simulink model "aes_impl_decrypt_smc"  (R2015b)
settings: Solver=FixedStepDiscrete  SolverMode=SingleTasking  StartTime=0.0  StopTime=1000e-6  RelTol=1e-3
undefined symbols (not defined in the file): a, b, input_sample_rate
libraries: shlslibv1 x3018
(part 4 of 20)

== system aes_impl_decrypt_smc/Round12/Subsystem8 ==
  In1 : Inport
  In2 : Inport  Port=2
  In3 : Inport  Port=3
  In4 : Inport  Port=4
  In5 : Inport  Port=5
  In6 : Inport  Port=6
  In7 : Inport  Port=7
  In8 : Inport  Port=8
  In9 : Inport  Port=9
  In10 : Inport  Port=10
  In11 : Inport  Port=11
  In12 : Inport  Port=12
  In13 : Inport  Port=13
  In14 : Inport  Port=14
  In15 : Inport  Port=15
  In16 : Inport  Port=16
  Subsystem : Subsystem
  Subsystem1 : Subsystem
  Subsystem2 : Subsystem
  Subsystem3 : Subsystem
  Subsystem4 : Subsystem
  Subsystem5 : Subsystem
  Subsystem6 : Subsystem
  Subsystem7 : Subsystem
  Subsystem8 : Subsystem
  Out1 : Outport
  Out2 : Outport  Port=2
  Out3 : Outport  Port=3
  Out4 : Outport  Port=4
  Out5 : Outport  Port=5
  Out6 : Outport  Port=6
  Out7 : Outport  Port=7
  Out8 : Outport  Port=8
  Out9 : Outport  Port=9
  Out10 : Outport  Port=10
  Out11 : Outport  Port=11
  Out12 : Outport  Port=12
  Out13 : Outport  Port=13
  Out14 : Outport  Port=14
  Out15 : Outport  Port=15
  Out16 : Outport  Port=16
  wires:
  Subsystem4/3(Out3) -> Out3/1
  Subsystem4/4(Out4) -> Out4/1
  Subsystem1/1(Out1) -> Out5/1
  Subsystem1/2(Out2) -> Out6/1
  Subsystem1/3(Out3) -> Out7/1
  Subsystem1/4(Out4) -> Out8/1
  Subsystem2/3(Out3) -> Out11/1
  Subsystem2/2(Out2) -> Out10/1
  Subsystem2/1(Out1) -> Out9/1
  Subsystem2/4(Out4) -> Out12/1
  Subsystem3/3(Out3) -> Out15/1
  Subsystem3/2(Out2) -> Out14/1
  Subsystem3/1(Out1) -> Out13/1
  Subsystem/1(Out1) -> Subsystem4/1(In1)
  Subsystem/2(Out2) -> Subsystem4/2(In2)
  Subsystem/3(Out3) -> Subsystem4/3(In3)
  Subsystem/4(Out4) -> Subsystem4/4(In4)
  Subsystem/5(Out5) -> Subsystem1/1(In1)
  Subsystem/6(Out6) -> Subsystem1/2(In2)
  Subsystem/7(Out7) -> Subsystem1/3(In3)
  Subsystem/8(Out8) -> Subsystem1/4(In4)
  Subsystem/9(Out9) -> Subsystem2/1(In1)
  Subsystem/10(Out10) -> Subsystem2/2(In2)
  Subsystem/11(Out11) -> Subsystem2/3(In3)
  Subsystem/12(Out12) -> Subsystem2/4(In4)
  Subsystem/14(Out14) -> Subsystem3/2(In2)
  Subsystem4/1(Out1) -> Out1/1
  Subsystem4/2(Out2) -> Out2/1
  Subsystem3/4(Out4) -> Out16/1
  Subsystem/13(Out13) -> Subsystem3/1(In1)
  Subsystem/15(Out15) -> Subsystem3/3(In3)
  Subsystem/16(Out16) -> Subsystem3/4(In4)
  Subsystem5/2(Out18) -> Subsystem/2(In2)
  Subsystem5/1(Out17) -> Subsystem/1(In1)
  Subsystem5/3(Out19) -> Subsystem/3(In3)
  Subsystem5/4(Out20) -> Subsystem/4(In4)
  In1/1 -> Subsystem5/1(In17)
  In2/1 -> Subsystem5/2(In18)
  In3/1 -> Subsystem5/3(In19)
  In4/1 -> Subsystem5/4(In20)
  Subsystem6/2(Out18) -> Subsystem/6(In6)
  Subsystem6/1(Out17) -> Subsystem/5(In5)
  Subsystem6/3(Out19) -> Subsystem/7(In7)
  Subsystem6/4(Out20) -> Subsystem/8(In8)
  In5/1 -> Subsystem6/1(In17)
  In6/1 -> Subsystem6/2(In18)
  In7/1 -> Subsystem6/3(In19)
  In8/1 -> Subsystem6/4(In20)
  Subsystem7/2(Out18) -> Subsystem/10(In10)
  Subsystem7/1(Out17) -> Subsystem/9(In9)
  Subsystem7/3(Out19) -> Subsystem/11(In11)
  Subsystem7/4(Out20) -> Subsystem/12(In12)
  In9/1 -> Subsystem7/1(In17)
  In10/1 -> Subsystem7/2(In18)
  In11/1 -> Subsystem7/3(In19)
  In12/1 -> Subsystem7/4(In20)
  Subsystem8/2(Out18) -> Subsystem/14(In14)
  Subsystem8/1(Out17) -> Subsystem/13(In13)
  Subsystem8/3(Out19) -> Subsystem/15(In15)
  Subsystem8/4(Out20) -> Subsystem/16(In16)
  In13/1 -> Subsystem8/1(In17)
  In14/1 -> Subsystem8/2(In18)
  In15/1 -> Subsystem8/3(In19)
  In16/1 -> Subsystem8/4(In20)

== system aes_impl_decrypt_smc/Round13/Subsystem ==
  In1 : Inport
  In2 : Inport  Port=2
  In3 : Inport  Port=3
  In4 : Inport  Port=4
  In5 : Inport  Port=5
  In6 : Inport  Port=6
  In7 : Inport  Port=7
  In8 : Inport  Port=8
  In9 : Inport  Port=9
  In10 : Inport  Port=10
  In11 : Inport  Port=11
  In12 : Inport  Port=12
  In13 : Inport  Port=13
  In14 : Inport  Port=14
  In15 : Inport  Port=15
  In16 : Inport  Port=16
  In17 : Inport  Port=17
  In18 : Inport  Port=18
  In19 : Inport  Port=19
  In20 : Inport  Port=20
  In21 : Inport  Port=21
  In22 : Inport  Port=22
  In23 : Inport  Port=23
  In24 : Inport  Port=24
  In25 : Inport  Port=25
  In26 : Inport  Port=26
  In27 : Inport  Port=27
  In28 : Inport  Port=28
  In29 : Inport  Port=29
  In30 : Inport  Port=30
  In31 : Inport  Port=31
  In32 : Inport  Port=32
  Binary Logic{,1..15} (16 alike) : shlslibv1/Math Functions/Binary Logic  syn_binlog_exp=a^b  synBlockType=primitive  synLatency=0  synBlockId=13
  Out1 : Outport
  Out2 : Outport  Port=2
  Out3 : Outport  Port=3
  Out4 : Outport  Port=4
  Out5 : Outport  Port=5
  Out6 : Outport  Port=6
  Out7 : Outport  Port=7
  Out8 : Outport  Port=8
  Out9 : Outport  Port=9
  Out10 : Outport  Port=10
  Out11 : Outport  Port=11
  Out12 : Outport  Port=12
  Out13 : Outport  Port=13
  Out14 : Outport  Port=14
  Out15 : Outport  Port=15
  Out16 : Outport  Port=16
  wires:
  In9/1 -> Binary Logic8/1
  In11/1 -> Binary Logic10/1
  In8/1 -> Binary Logic7/1
  In16/1 -> Binary Logic15/1
  In3/1 -> Binary Logic2/1
  In12/1 -> Binary Logic11/1
  In10/1 -> Binary Logic9/1
  In13/1 -> Binary Logic12/1
  In15/1 -> Binary Logic14/1
  In14/1 -> Binary Logic13/1
  In7/1 -> Binary Logic6/1
  In6/1 -> Binary Logic5/1
  Binary Logic/1 -> Out1/1
  In4/1 -> Binary Logic3/1
  In5/1 -> Binary Logic4/1
  In2/1 -> Binary Logic1/1
  In18/1 -> Binary Logic1/2
  In19/1 -> Binary Logic2/2
  In20/1 -> Binary Logic3/2
  In21/1 -> Binary Logic4/2
  In22/1 -> Binary Logic5/2
  In23/1 -> Binary Logic6/2
  In24/1 -> Binary Logic7/2
  In25/1 -> Binary Logic8/2
  In26/1 -> Binary Logic9/2
  In27/1 -> Binary Logic10/2
  In28/1 -> Binary Logic11/2
  In29/1 -> Binary Logic12/2
  In30/1 -> Binary Logic13/2
  In31/1 -> Binary Logic14/2
  In32/1 -> Binary Logic15/2
  In1/1 -> Binary Logic/1
  In17/1 -> Binary Logic/2
  Binary Logic1/1 -> Out2/1
  Binary Logic2/1 -> Out3/1
  Binary Logic3/1 -> Out4/1
  Binary Logic4/1 -> Out5/1
  Binary Logic5/1 -> Out6/1
  Binary Logic6/1 -> Out7/1
  Binary Logic7/1 -> Out8/1
  Binary Logic8/1 -> Out9/1
  Binary Logic9/1 -> Out10/1
  Binary Logic15/1 -> Out16/1
  Binary Logic14/1 -> Out15/1
  Binary Logic13/1 -> Out14/1
  Binary Logic12/1 -> Out13/1
  Binary Logic11/1 -> Out12/1
  Binary Logic10/1 -> Out11/1

== system aes_impl_decrypt_smc/Round13/Subsystem8 ==
  In1 : Inport
  In2 : Inport  Port=2
  In3 : Inport  Port=3
  In4 : Inport  Port=4
  In5 : Inport  Port=5
  In6 : Inport  Port=6
  In7 : Inport  Port=7
  In8 : Inport  Port=8
  In9 : Inport  Port=9
  In10 : Inport  Port=10
  In11 : Inport  Port=11
  In12 : Inport  Port=12
  In13 : Inport  Port=13
  In14 : Inport  Port=14
  In15 : Inport  Port=15
  In16 : Inport  Port=16
  Subsystem : Subsystem
  Subsystem1 : Subsystem
  Subsystem2 : Subsystem
  Subsystem3 : Subsystem
  Subsystem4 : Subsystem
  Out1 : Outport
  Out2 : Outport  Port=2
  Out3 : Outport  Port=3
  Out4 : Outport  Port=4
  Out5 : Outport  Port=5
  Out6 : Outport  Port=6
  Out7 : Outport  Port=7
  Out8 : Outport  Port=8
  Out9 : Outport  Port=9
  Out10 : Outport  Port=10
  Out11 : Outport  Port=11
  Out12 : Outport  Port=12
  Out13 : Outport  Port=13
  Out14 : Outport  Port=14
  Out15 : Outport  Port=15
  Out16 : Outport  Port=16
  wires:
  Subsystem4/3(Out3) -> Out3/1
  Subsystem4/4(Out4) -> Out4/1
  Subsystem1/1(Out1) -> Out5/1
  Subsystem1/2(Out2) -> Out6/1
  Subsystem1/3(Out3) -> Out7/1
  Subsystem1/4(Out4) -> Out8/1
  Subsystem2/3(Out3) -> Out11/1
  Subsystem2/2(Out2) -> Out10/1
  Subsystem2/1(Out1) -> Out9/1
  Subsystem2/4(Out4) -> Out12/1
  Subsystem3/3(Out3) -> Out15/1
  Subsystem3/2(Out2) -> Out14/1
  Subsystem3/1(Out1) -> Out13/1
  In1/1 -> Subsystem/1(In1)
  In2/1 -> Subsystem/2(In2)
  In3/1 -> Subsystem/3(In3)
  In4/1 -> Subsystem/4(In4)
  In5/1 -> Subsystem/5(In5)
  In6/1 -> Subsystem/6(In6)
  In7/1 -> Subsystem/7(In7)
  In8/1 -> Subsystem/8(In8)
  In9/1 -> Subsystem/9(In9)
  In10/1 -> Subsystem/10(In10)
  In11/1 -> Subsystem/11(In11)
  In12/1 -> Subsystem/12(In12)
  In13/1 -> Subsystem/13(In13)
  In14/1 -> Subsystem/14(In14)
  In15/1 -> Subsystem/15(In15)
  In16/1 -> Subsystem/16(In16)
  Subsystem/1(Out1) -> Subsystem4/1(In1)
  Subsystem/2(Out2) -> Subsystem4/2(In2)
  Subsystem/3(Out3) -> Subsystem4/3(In3)
  Subsystem/4(Out4) -> Subsystem4/4(In4)
  Subsystem/5(Out5) -> Subsystem1/1(In1)
  Subsystem/6(Out6) -> Subsystem1/2(In2)
  Subsystem/7(Out7) -> Subsystem1/3(In3)
  Subsystem/8(Out8) -> Subsystem1/4(In4)
  Subsystem/9(Out9) -> Subsystem2/1(In1)
  Subsystem/10(Out10) -> Subsystem2/2(In2)
  Subsystem/11(Out11) -> Subsystem2/3(In3)
  Subsystem/12(Out12) -> Subsystem2/4(In4)
  Subsystem/14(Out14) -> Subsystem3/2(In2)
  Subsystem4/1(Out1) -> Out1/1
  Subsystem4/2(Out2) -> Out2/1
  Subsystem3/4(Out4) -> Out16/1
  Subsystem/13(Out13) -> Subsystem3/1(In1)
  Subsystem/15(Out15) -> Subsystem3/3(In3)
  Subsystem/16(Out16) -> Subsystem3/4(In4)

== system aes_impl_decrypt_smc/Round14/Subsystem ==
  In1 : Inport
  In2 : Inport  Port=2
  In3 : Inport  Port=3
  In4 : Inport  Port=4
  In5 : Inport  Port=5
  In6 : Inport  Port=6
  In7 : Inport  Port=7
  In8 : Inport  Port=8
  In9 : Inport  Port=9
  In10 : Inport  Port=10
  In11 : Inport  Port=11
  In12 : Inport  Port=12
  In13 : Inport  Port=13
  In14 : Inport  Port=14
  In15 : Inport  Port=15
  In16 : Inport  Port=16
  In17 : Inport  Port=17
  In18 : Inport  Port=18
  In19 : Inport  Port=19
  In20 : Inport  Port=20
  In21 : Inport  Port=21
  In22 : Inport  Port=22
  In23 : Inport  Port=23
  In24 : Inport  Port=24
  In25 : Inport  Port=25
  In26 : Inport  Port=26
  In27 : Inport  Port=27
  In28 : Inport  Port=28
  In29 : Inport  Port=29
  In30 : Inport  Port=30
  In31 : Inport  Port=31
  In32 : Inport  Port=32
  Binary Logic{,1..15} (16 alike) : shlslibv1/Math Functions/Binary Logic  syn_binlog_exp=a^b  synBlockType=primitive  synLatency=0  synBlockId=13
  Out1 : Outport
  Out2 : Outport  Port=2
  Out3 : Outport  Port=3
  Out4 : Outport  Port=4
  Out5 : Outport  Port=5
  Out6 : Outport  Port=6
  Out7 : Outport  Port=7
  Out8 : Outport  Port=8
  Out9 : Outport  Port=9
  Out10 : Outport  Port=10
  Out11 : Outport  Port=11
  Out12 : Outport  Port=12
  Out13 : Outport  Port=13
  Out14 : Outport  Port=14
  Out15 : Outport  Port=15
  Out16 : Outport  Port=16
  wires:
  In9/1 -> Binary Logic8/1
  In11/1 -> Binary Logic10/1
  In8/1 -> Binary Logic7/1
  In16/1 -> Binary Logic15/1
  In3/1 -> Binary Logic2/1
  In12/1 -> Binary Logic11/1
  In10/1 -> Binary Logic9/1
  In13/1 -> Binary Logic12/1
  In15/1 -> Binary Logic14/1
  In14/1 -> Binary Logic13/1
  In7/1 -> Binary Logic6/1
  In6/1 -> Binary Logic5/1
  Binary Logic/1 -> Out1/1
  In4/1 -> Binary Logic3/1
  In5/1 -> Binary Logic4/1
  In2/1 -> Binary Logic1/1
  In18/1 -> Binary Logic1/2
  In19/1 -> Binary Logic2/2
  In20/1 -> Binary Logic3/2
  In21/1 -> Binary Logic4/2
  In22/1 -> Binary Logic5/2
  In23/1 -> Binary Logic6/2
  In24/1 -> Binary Logic7/2
  In25/1 -> Binary Logic8/2
  In26/1 -> Binary Logic9/2
  In27/1 -> Binary Logic10/2
  In28/1 -> Binary Logic11/2
  In29/1 -> Binary Logic12/2
  In30/1 -> Binary Logic13/2
  In31/1 -> Binary Logic14/2
  In32/1 -> Binary Logic15/2
  In1/1 -> Binary Logic/1
  In17/1 -> Binary Logic/2
  Binary Logic1/1 -> Out2/1
  Binary Logic2/1 -> Out3/1
  Binary Logic3/1 -> Out4/1
  Binary Logic4/1 -> Out5/1
  Binary Logic5/1 -> Out6/1
  Binary Logic6/1 -> Out7/1
  Binary Logic7/1 -> Out8/1
  Binary Logic8/1 -> Out9/1
  Binary Logic9/1 -> Out10/1
  Binary Logic15/1 -> Out16/1
  Binary Logic14/1 -> Out15/1
  Binary Logic13/1 -> Out14/1
  Binary Logic12/1 -> Out13/1
  Binary Logic11/1 -> Out12/1
  Binary Logic10/1 -> Out11/1

== system aes_impl_decrypt_smc/Round14/Subsystem8 ==
  In1 : Inport
  In2 : Inport  Port=2
  In3 : Inport  Port=3
  In4 : Inport  Port=4
  In5 : Inport  Port=5
  In6 : Inport  Port=6
  In7 : Inport  Port=7
  In8 : Inport  Port=8
  In9 : Inport  Port=9
  In10 : Inport  Port=10
  In11 : Inport  Port=11
  In12 : Inport  Port=12
  In13 : Inport  Port=13
  In14 : Inport  Port=14
  In15 : Inport  Port=15
  In16 : Inport  Port=16
  Subsystem : Subsystem
  Subsystem1 : Subsystem
  Subsystem2 : Subsystem
  Subsystem3 : Subsystem
  Subsystem4 : Subsystem
  Subsystem5 : Subsystem
  Subsystem6 : Subsystem
  Subsystem7 : Subsystem
  Subsystem8 : Subsystem
  Out1 : Outport
  Out2 : Outport  Port=2
  Out3 : Outport  Port=3
  Out4 : Outport  Port=4
  Out5 : Outport  Port=5
  Out6 : Outport  Port=6
  Out7 : Outport  Port=7
  Out8 : Outport  Port=8
  Out9 : Outport  Port=9
  Out10 : Outport  Port=10
  Out11 : Outport  Port=11
  Out12 : Outport  Port=12
  Out13 : Outport  Port=13
  Out14 : Outport  Port=14
  Out15 : Outport  Port=15
  Out16 : Outport  Port=16
  wires:
  Subsystem4/3(Out3) -> Out3/1
  Subsystem4/4(Out4) -> Out4/1
  Subsystem1/1(Out1) -> Out5/1
  Subsystem1/2(Out2) -> Out6/1
  Subsystem1/3(Out3) -> Out7/1
  Subsystem1/4(Out4) -> Out8/1
  Subsystem2/3(Out3) -> Out11/1
  Subsystem2/2(Out2) -> Out10/1
  Subsystem2/1(Out1) -> Out9/1
  Subsystem2/4(Out4) -> Out12/1
  Subsystem3/3(Out3) -> Out15/1
  Subsystem3/2(Out2) -> Out14/1
  Subsystem3/1(Out1) -> Out13/1
  Subsystem/1(Out1) -> Subsystem4/1(In1)
  Subsystem/2(Out2) -> Subsystem4/2(In2)
  Subsystem/3(Out3) -> Subsystem4/3(In3)
  Subsystem/4(Out4) -> Subsystem4/4(In4)
  Subsystem/5(Out5) -> Subsystem1/1(In1)
  Subsystem/6(Out6) -> Subsystem1/2(In2)
  Subsystem/7(Out7) -> Subsystem1/3(In3)
  Subsystem/8(Out8) -> Subsystem1/4(In4)
  Subsystem/9(Out9) -> Subsystem2/1(In1)
  Subsystem/10(Out10) -> Subsystem2/2(In2)
  Subsystem/11(Out11) -> Subsystem2/3(In3)
  Subsystem/12(Out12) -> Subsystem2/4(In4)
  Subsystem/14(Out14) -> Subsystem3/2(In2)
  Subsystem4/1(Out1) -> Out1/1
  Subsystem4/2(Out2) -> Out2/1
  Subsystem3/4(Out4) -> Out16/1
  Subsystem/13(Out13) -> Subsystem3/1(In1)
  Subsystem/15(Out15) -> Subsystem3/3(In3)
  Subsystem/16(Out16) -> Subsystem3/4(In4)
  Subsystem5/2(Out18) -> Subsystem/2(In2)
  Subsystem5/1(Out17) -> Subsystem/1(In1)
  Subsystem5/3(Out19) -> Subsystem/3(In3)
  Subsystem5/4(Out20) -> Subsystem/4(In4)
  In1/1 -> Subsystem5/1(In17)
  In2/1 -> Subsystem5/2(In18)
  In3/1 -> Subsystem5/3(In19)
  In4/1 -> Subsystem5/4(In20)
  Subsystem6/2(Out18) -> Subsystem/6(In6)
  Subsystem6/1(Out17) -> Subsystem/5(In5)
  Subsystem6/3(Out19) -> Subsystem/7(In7)
  Subsystem6/4(Out20) -> Subsystem/8(In8)
  In5/1 -> Subsystem6/1(In17)
  In6/1 -> Subsystem6/2(In18)
  In7/1 -> Subsystem6/3(In19)
  In8/1 -> Subsystem6/4(In20)
  Subsystem7/2(Out18) -> Subsystem/10(In10)
  Subsystem7/1(Out17) -> Subsystem/9(In9)
  Subsystem7/3(Out19) -> Subsystem/11(In11)
  Subsystem7/4(Out20) -> Subsystem/12(In12)
  In9/1 -> Subsystem7/1(In17)
  In10/1 -> Subsystem7/2(In18)
  In11/1 -> Subsystem7/3(In19)
  In12/1 -> Subsystem7/4(In20)
  Subsystem8/2(Out18) -> Subsystem/14(In14)
  Subsystem8/1(Out17) -> Subsystem/13(In13)
  Subsystem8/3(Out19) -> Subsystem/15(In15)
  Subsystem8/4(Out20) -> Subsystem/16(In16)
  In13/1 -> Subsystem8/1(In17)
  In14/1 -> Subsystem8/2(In18)
  In15/1 -> Subsystem8/3(In19)
  In16/1 -> Subsystem8/4(In20)

== system aes_impl_decrypt_smc/Round15/Subsystem ==
  In1 : Inport
  In2 : Inport  Port=2
  In3 : Inport  Port=3
  In4 : Inport  Port=4
  In5 : Inport  Port=5
  In6 : Inport  Port=6
  In7 : Inport  Port=7
  In8 : Inport  Port=8
  In9 : Inport  Port=9
  In10 : Inport  Port=10
  In11 : Inport  Port=11
  In12 : Inport  Port=12
  In13 : Inport  Port=13
  In14 : Inport  Port=14
  In15 : Inport  Port=15
  In16 : Inport  Port=16
  In17 : Inport  Port=17
  In18 : Inport  Port=18
  In19 : Inport  Port=19
  In20 : Inport  Port=20
  In21 : Inport  Port=21
  In22 : Inport  Port=22
  In23 : Inport  Port=23
  In24 : Inport  Port=24
  In25 : Inport  Port=25
  In26 : Inport  Port=26
  In27 : Inport  Port=27
  In28 : Inport  Port=28
  In29 : Inport  Port=29
  In30 : Inport  Port=30
  In31 : Inport  Port=31
  In32 : Inport  Port=32
  Binary Logic{,1..15} (16 alike) : shlslibv1/Math Functions/Binary Logic  syn_binlog_exp=a^b  synBlockType=primitive  synLatency=0  synBlockId=13
  Out1 : Outport
  Out2 : Outport  Port=2
  Out3 : Outport  Port=3
  Out4 : Outport  Port=4
  Out5 : Outport  Port=5
  Out6 : Outport  Port=6
  Out7 : Outport  Port=7
  Out8 : Outport  Port=8
  Out9 : Outport  Port=9
  Out10 : Outport  Port=10
  Out11 : Outport  Port=11
  Out12 : Outport  Port=12
  Out13 : Outport  Port=13
  Out14 : Outport  Port=14
  Out15 : Outport  Port=15
  Out16 : Outport  Port=16
  wires:
  In9/1 -> Binary Logic8/1
  In11/1 -> Binary Logic10/1
  In8/1 -> Binary Logic7/1
  In16/1 -> Binary Logic15/1
  In3/1 -> Binary Logic2/1
  In12/1 -> Binary Logic11/1
  In10/1 -> Binary Logic9/1
  In13/1 -> Binary Logic12/1
  In15/1 -> Binary Logic14/1
  In14/1 -> Binary Logic13/1
  In7/1 -> Binary Logic6/1
  In6/1 -> Binary Logic5/1
  Binary Logic/1 -> Out1/1
  In4/1 -> Binary Logic3/1
  In5/1 -> Binary Logic4/1
  In2/1 -> Binary Logic1/1
  In18/1 -> Binary Logic1/2
  In19/1 -> Binary Logic2/2
  In20/1 -> Binary Logic3/2
  In21/1 -> Binary Logic4/2
  In22/1 -> Binary Logic5/2
  In23/1 -> Binary Logic6/2
  In24/1 -> Binary Logic7/2
  In25/1 -> Binary Logic8/2
  In26/1 -> Binary Logic9/2
  In27/1 -> Binary Logic10/2
  In28/1 -> Binary Logic11/2
  In29/1 -> Binary Logic12/2
  In30/1 -> Binary Logic13/2
  In31/1 -> Binary Logic14/2
  In32/1 -> Binary Logic15/2
  In1/1 -> Binary Logic/1
  In17/1 -> Binary Logic/2
  Binary Logic1/1 -> Out2/1
  Binary Logic2/1 -> Out3/1
  Binary Logic3/1 -> Out4/1
  Binary Logic4/1 -> Out5/1
  Binary Logic5/1 -> Out6/1
  Binary Logic6/1 -> Out7/1
  Binary Logic7/1 -> Out8/1
  Binary Logic8/1 -> Out9/1
  Binary Logic9/1 -> Out10/1
  Binary Logic15/1 -> Out16/1
  Binary Logic14/1 -> Out15/1
  Binary Logic13/1 -> Out14/1
  Binary Logic12/1 -> Out13/1
  Binary Logic11/1 -> Out12/1
  Binary Logic10/1 -> Out11/1

== system aes_impl_decrypt_smc/Round15/Subsystem8 ==
  In1 : Inport
  In2 : Inport  Port=2
  In3 : Inport  Port=3
  In4 : Inport  Port=4
  In5 : Inport  Port=5
  In6 : Inport  Port=6
  In7 : Inport  Port=7
  In8 : Inport  Port=8
  In9 : Inport  Port=9
  In10 : Inport  Port=10
  In11 : Inport  Port=11
  In12 : Inport  Port=12
  In13 : Inport  Port=13
  In14 : Inport  Port=14
  In15 : Inport  Port=15
  In16 : Inport  Port=16
  Subsystem : Subsystem
  Subsystem1 : Subsystem
  Subsystem2 : Subsystem
  Subsystem3 : Subsystem
  Subsystem4 : Subsystem
  Subsystem5 : Subsystem
  Subsystem6 : Subsystem
  Subsystem7 : Subsystem
  Subsystem8 : Subsystem
  Out1 : Outport
  Out2 : Outport  Port=2
  Out3 : Outport  Port=3
  Out4 : Outport  Port=4
  Out5 : Outport  Port=5
  Out6 : Outport  Port=6
  Out7 : Outport  Port=7
  Out8 : Outport  Port=8
  Out9 : Outport  Port=9
  Out10 : Outport  Port=10
  Out11 : Outport  Port=11
  Out12 : Outport  Port=12
  Out13 : Outport  Port=13
  Out14 : Outport  Port=14
  Out15 : Outport  Port=15
  Out16 : Outport  Port=16
  wires:
  Subsystem4/3(Out3) -> Out3/1
  Subsystem4/4(Out4) -> Out4/1
  Subsystem1/1(Out1) -> Out5/1
  Subsystem1/2(Out2) -> Out6/1
  Subsystem1/3(Out3) -> Out7/1
  Subsystem1/4(Out4) -> Out8/1
  Subsystem2/3(Out3) -> Out11/1
  Subsystem2/2(Out2) -> Out10/1
  Subsystem2/1(Out1) -> Out9/1
  Subsystem2/4(Out4) -> Out12/1
  Subsystem3/3(Out3) -> Out15/1
  Subsystem3/2(Out2) -> Out14/1
  Subsystem3/1(Out1) -> Out13/1
  Subsystem/1(Out1) -> Subsystem4/1(In1)
  Subsystem/2(Out2) -> Subsystem4/2(In2)
  Subsystem/3(Out3) -> Subsystem4/3(In3)
  Subsystem/4(Out4) -> Subsystem4/4(In4)
  Subsystem/5(Out5) -> Subsystem1/1(In1)
  Subsystem/6(Out6) -> Subsystem1/2(In2)
  Subsystem/7(Out7) -> Subsystem1/3(In3)
  Subsystem/8(Out8) -> Subsystem1/4(In4)
  Subsystem/9(Out9) -> Subsystem2/1(In1)
  Subsystem/10(Out10) -> Subsystem2/2(In2)
  Subsystem/11(Out11) -> Subsystem2/3(In3)
  Subsystem/12(Out12) -> Subsystem2/4(In4)
  Subsystem/14(Out14) -> Subsystem3/2(In2)
  Subsystem4/1(Out1) -> Out1/1
  Subsystem4/2(Out2) -> Out2/1
  Subsystem3/4(Out4) -> Out16/1
  Subsystem/13(Out13) -> Subsystem3/1(In1)
  Subsystem/15(Out15) -> Subsystem3/3(In3)
  Subsystem/16(Out16) -> Subsystem3/4(In4)
  Subsystem5/2(Out18) -> Subsystem/2(In2)
  Subsystem5/1(Out17) -> Subsystem/1(In1)
  Subsystem5/3(Out19) -> Subsystem/3(In3)
  Subsystem5/4(Out20) -> Subsystem/4(In4)
  In1/1 -> Subsystem5/1(In17)
  In2/1 -> Subsystem5/2(In18)
  In3/1 -> Subsystem5/3(In19)
  In4/1 -> Subsystem5/4(In20)
  Subsystem6/2(Out18) -> Subsystem/6(In6)
  Subsystem6/1(Out17) -> Subsystem/5(In5)
  Subsystem6/3(Out19) -> Subsystem/7(In7)
  Subsystem6/4(Out20) -> Subsystem/8(In8)
  In5/1 -> Subsystem6/1(In17)
  In6/1 -> Subsystem6/2(In18)
  In7/1 -> Subsystem6/3(In19)
  In8/1 -> Subsystem6/4(In20)
  Subsystem7/2(Out18) -> Subsystem/10(In10)
  Subsystem7/1(Out17) -> Subsystem/9(In9)
  Subsystem7/3(Out19) -> Subsystem/11(In11)
  Subsystem7/4(Out20) -> Subsystem/12(In12)
  In9/1 -> Subsystem7/1(In17)
  In10/1 -> Subsystem7/2(In18)
  In11/1 -> Subsystem7/3(In19)
  In12/1 -> Subsystem7/4(In20)
  Subsystem8/2(Out18) -> Subsystem/14(In14)
  Subsystem8/1(Out17) -> Subsystem/13(In13)
  Subsystem8/3(Out19) -> Subsystem/15(In15)
  Subsystem8/4(Out20) -> Subsystem/16(In16)
  In13/1 -> Subsystem8/1(In17)
  In14/1 -> Subsystem8/2(In18)
  In15/1 -> Subsystem8/3(In19)
  In16/1 -> Subsystem8/4(In20)

== system aes_impl_decrypt_smc/Round16/Subsystem ==
  In1 : Inport
  In2 : Inport  Port=2
  In3 : Inport  Port=3
  In4 : Inport  Port=4
  In5 : Inport  Port=5
  In6 : Inport  Port=6
  In7 : Inport  Port=7
  In8 : Inport  Port=8
  In9 : Inport  Port=9
  In10 : Inport  Port=10
  In11 : Inport  Port=11
  In12 : Inport  Port=12
  In13 : Inport  Port=13
  In14 : Inport  Port=14
  In15 : Inport  Port=15
  In16 : Inport  Port=16
  In17 : Inport  Port=17
  In18 : Inport  Port=18
  In19 : Inport  Port=19
  In20 : Inport  Port=20
  In21 : Inport  Port=21
  In22 : Inport  Port=22
  In23 : Inport  Port=23
  In24 : Inport  Port=24
  In25 : Inport  Port=25
  In26 : Inport  Port=26
  In27 : Inport  Port=27
  In28 : Inport  Port=28
  In29 : Inport  Port=29
  In30 : Inport  Port=30
  In31 : Inport  Port=31
  In32 : Inport  Port=32
  Binary Logic{,1..15} (16 alike) : shlslibv1/Math Functions/Binary Logic  syn_binlog_exp=a^b  synBlockType=primitive  synLatency=0  synBlockId=13
  Out1 : Outport
  Out2 : Outport  Port=2
  Out3 : Outport  Port=3
  Out4 : Outport  Port=4
  Out5 : Outport  Port=5
  Out6 : Outport  Port=6
  Out7 : Outport  Port=7
  Out8 : Outport  Port=8
  Out9 : Outport  Port=9
  Out10 : Outport  Port=10
  Out11 : Outport  Port=11
  Out12 : Outport  Port=12
  Out13 : Outport  Port=13
  Out14 : Outport  Port=14
  Out15 : Outport  Port=15
  Out16 : Outport  Port=16
  wires:
  In9/1 -> Binary Logic8/1
  In11/1 -> Binary Logic10/1
  In8/1 -> Binary Logic7/1
  In16/1 -> Binary Logic15/1
  In3/1 -> Binary Logic2/1
  In12/1 -> Binary Logic11/1
  In10/1 -> Binary Logic9/1
  In13/1 -> Binary Logic12/1
  In15/1 -> Binary Logic14/1
  In14/1 -> Binary Logic13/1
  In7/1 -> Binary Logic6/1
  In6/1 -> Binary Logic5/1
  Binary Logic/1 -> Out1/1
  In4/1 -> Binary Logic3/1
  In5/1 -> Binary Logic4/1
  In2/1 -> Binary Logic1/1
  In18/1 -> Binary Logic1/2
  In19/1 -> Binary Logic2/2
  In20/1 -> Binary Logic3/2
  In21/1 -> Binary Logic4/2
  In22/1 -> Binary Logic5/2
  In23/1 -> Binary Logic6/2
  In24/1 -> Binary Logic7/2
  In25/1 -> Binary Logic8/2
  In26/1 -> Binary Logic9/2
  In27/1 -> Binary Logic10/2
  In28/1 -> Binary Logic11/2
  In29/1 -> Binary Logic12/2
  In30/1 -> Binary Logic13/2
  In31/1 -> Binary Logic14/2
  In32/1 -> Binary Logic15/2
  In1/1 -> Binary Logic/1
  In17/1 -> Binary Logic/2
  Binary Logic1/1 -> Out2/1
  Binary Logic2/1 -> Out3/1
  Binary Logic3/1 -> Out4/1
  Binary Logic4/1 -> Out5/1
  Binary Logic5/1 -> Out6/1
  Binary Logic6/1 -> Out7/1
  Binary Logic7/1 -> Out8/1
  Binary Logic8/1 -> Out9/1
  Binary Logic9/1 -> Out10/1
  Binary Logic15/1 -> Out16/1
  Binary Logic14/1 -> Out15/1
  Binary Logic13/1 -> Out14/1
  Binary Logic12/1 -> Out13/1
  Binary Logic11/1 -> Out12/1
  Binary Logic10/1 -> Out11/1

== system aes_impl_decrypt_smc/Round16/Subsystem8 ==
  In1 : Inport
  In2 : Inport  Port=2
  In3 : Inport  Port=3
  In4 : Inport  Port=4
  In5 : Inport  Port=5
  In6 : Inport  Port=6
  In7 : Inport  Port=7
  In8 : Inport  Port=8
  In9 : Inport  Port=9
  In10 : Inport  Port=10
  In11 : Inport  Port=11
  In12 : Inport  Port=12
  In13 : Inport  Port=13
  In14 : Inport  Port=14
  In15 : Inport  Port=15
  In16 : Inport  Port=16
  Subsystem : Subsystem
  Subsystem1 : Subsystem
  Subsystem2 : Subsystem
  Subsystem3 : Subsystem
  Subsystem4 : Subsystem
  Subsystem5 : Subsystem
  Subsystem6 : Subsystem
  Subsystem7 : Subsystem
  Subsystem8 : Subsystem
  Out1 : Outport
  Out2 : Outport  Port=2
  Out3 : Outport  Port=3
  Out4 : Outport  Port=4
  Out5 : Outport  Port=5
  Out6 : Outport  Port=6
  Out7 : Outport  Port=7
  Out8 : Outport  Port=8
  Out9 : Outport  Port=9
  Out10 : Outport  Port=10
  Out11 : Outport  Port=11
  Out12 : Outport  Port=12
  Out13 : Outport  Port=13
  Out14 : Outport  Port=14
  Out15 : Outport  Port=15
  Out16 : Outport  Port=16
  wires:
  Subsystem4/3(Out3) -> Out3/1
  Subsystem4/4(Out4) -> Out4/1
  Subsystem1/1(Out1) -> Out5/1
  Subsystem1/2(Out2) -> Out6/1
  Subsystem1/3(Out3) -> Out7/1
  Subsystem1/4(Out4) -> Out8/1
  Subsystem2/3(Out3) -> Out11/1
  Subsystem2/2(Out2) -> Out10/1
  Subsystem2/1(Out1) -> Out9/1
  Subsystem2/4(Out4) -> Out12/1
  Subsystem3/3(Out3) -> Out15/1
  Subsystem3/2(Out2) -> Out14/1
  Subsystem3/1(Out1) -> Out13/1
  Subsystem/1(Out1) -> Subsystem4/1(In1)
  Subsystem/2(Out2) -> Subsystem4/2(In2)
  Subsystem/3(Out3) -> Subsystem4/3(In3)
  Subsystem/4(Out4) -> Subsystem4/4(In4)
  Subsystem/5(Out5) -> Subsystem1/1(In1)
  Subsystem/6(Out6) -> Subsystem1/2(In2)
  Subsystem/7(Out7) -> Subsystem1/3(In3)
  Subsystem/8(Out8) -> Subsystem1/4(In4)
  Subsystem/9(Out9) -> Subsystem2/1(In1)
  Subsystem/10(Out10) -> Subsystem2/2(In2)
  Subsystem/11(Out11) -> Subsystem2/3(In3)
  Subsystem/12(Out12) -> Subsystem2/4(In4)
  Subsystem/14(Out14) -> Subsystem3/2(In2)
  Subsystem4/1(Out1) -> Out1/1
  Subsystem4/2(Out2) -> Out2/1
  Subsystem3/4(Out4) -> Out16/1
  Subsystem/13(Out13) -> Subsystem3/1(In1)
  Subsystem/15(Out15) -> Subsystem3/3(In3)
  Subsystem/16(Out16) -> Subsystem3/4(In4)
  Subsystem5/2(Out18) -> Subsystem/2(In2)
  Subsystem5/1(Out17) -> Subsystem/1(In1)
  Subsystem5/3(Out19) -> Subsystem/3(In3)
  Subsystem5/4(Out20) -> Subsystem/4(In4)
  In1/1 -> Subsystem5/1(In17)
  In2/1 -> Subsystem5/2(In18)
  In3/1 -> Subsystem5/3(In19)
  In4/1 -> Subsystem5/4(In20)
  Subsystem6/2(Out18) -> Subsystem/6(In6)
  Subsystem6/1(Out17) -> Subsystem/5(In5)
  Subsystem6/3(Out19) -> Subsystem/7(In7)
  Subsystem6/4(Out20) -> Subsystem/8(In8)
  In5/1 -> Subsystem6/1(In17)
  In6/1 -> Subsystem6/2(In18)
  In7/1 -> Subsystem6/3(In19)
  In8/1 -> Subsystem6/4(In20)
  Subsystem7/2(Out18) -> Subsystem/10(In10)
  Subsystem7/1(Out17) -> Subsystem/9(In9)
  Subsystem7/3(Out19) -> Subsystem/11(In11)
  Subsystem7/4(Out20) -> Subsystem/12(In12)
  In9/1 -> Subsystem7/1(In17)
  In10/1 -> Subsystem7/2(In18)
  In11/1 -> Subsystem7/3(In19)
  In12/1 -> Subsystem7/4(In20)
  Subsystem8/2(Out18) -> Subsystem/14(In14)
  Subsystem8/1(Out17) -> Subsystem/13(In13)
  Subsystem8/3(Out19) -> Subsystem/15(In15)
  Subsystem8/4(Out20) -> Subsystem/16(In16)
  In13/1 -> Subsystem8/1(In17)
  In14/1 -> Subsystem8/2(In18)
  In15/1 -> Subsystem8/3(In19)
  In16/1 -> Subsystem8/4(In20)

== system aes_impl_decrypt_smc/Round17/Subsystem ==
  In1 : Inport
  In2 : Inport  Port=2
  In3 : Inport  Port=3
  In4 : Inport  Port=4
  In5 : Inport  Port=5
  In6 : Inport  Port=6
  In7 : Inport  Port=7
  In8 : Inport  Port=8
  In9 : Inport  Port=9
  In10 : Inport  Port=10
  In11 : Inport  Port=11
  In12 : Inport  Port=12
  In13 : Inport  Port=13
  In14 : Inport  Port=14
  In15 : Inport  Port=15
  In16 : Inport  Port=16
  In17 : Inport  Port=17
  In18 : Inport  Port=18
  In19 : Inport  Port=19
  In20 : Inport  Port=20
  In21 : Inport  Port=21
  In22 : Inport  Port=22
  In23 : Inport  Port=23
  In24 : Inport  Port=24
  In25 : Inport  Port=25
  In26 : Inport  Port=26
  In27 : Inport  Port=27
  In28 : Inport  Port=28
  In29 : Inport  Port=29
  In30 : Inport  Port=30
  In31 : Inport  Port=31
  In32 : Inport  Port=32
  Binary Logic{,1..15} (16 alike) : shlslibv1/Math Functions/Binary Logic  syn_binlog_exp=a^b  synBlockType=primitive  synLatency=0  synBlockId=13
  Out1 : Outport
  Out2 : Outport  Port=2
  Out3 : Outport  Port=3
  Out4 : Outport  Port=4
  Out5 : Outport  Port=5
  Out6 : Outport  Port=6
  Out7 : Outport  Port=7
  Out8 : Outport  Port=8
  Out9 : Outport  Port=9
  Out10 : Outport  Port=10
  Out11 : Outport  Port=11
  Out12 : Outport  Port=12
  Out13 : Outport  Port=13
  Out14 : Outport  Port=14
  Out15 : Outport  Port=15
  Out16 : Outport  Port=16
  wires:
  In9/1 -> Binary Logic8/1
  In11/1 -> Binary Logic10/1
  In8/1 -> Binary Logic7/1
  In16/1 -> Binary Logic15/1
  In3/1 -> Binary Logic2/1
  In12/1 -> Binary Logic11/1
  In10/1 -> Binary Logic9/1
  In13/1 -> Binary Logic12/1
  In15/1 -> Binary Logic14/1
  In14/1 -> Binary Logic13/1
  In7/1 -> Binary Logic6/1
  In6/1 -> Binary Logic5/1
  Binary Logic/1 -> Out1/1
  In4/1 -> Binary Logic3/1
  In5/1 -> Binary Logic4/1
  In2/1 -> Binary Logic1/1
  In18/1 -> Binary Logic1/2
  In19/1 -> Binary Logic2/2
  In20/1 -> Binary Logic3/2
  In21/1 -> Binary Logic4/2
  In22/1 -> Binary Logic5/2
  In23/1 -> Binary Logic6/2
  In24/1 -> Binary Logic7/2
  In25/1 -> Binary Logic8/2
  In26/1 -> Binary Logic9/2
  In27/1 -> Binary Logic10/2
  In28/1 -> Binary Logic11/2
  In29/1 -> Binary Logic12/2
  In30/1 -> Binary Logic13/2
  In31/1 -> Binary Logic14/2
  In32/1 -> Binary Logic15/2
  In1/1 -> Binary Logic/1
  In17/1 -> Binary Logic/2
  Binary Logic1/1 -> Out2/1
  Binary Logic2/1 -> Out3/1
  Binary Logic3/1 -> Out4/1
  Binary Logic4/1 -> Out5/1
  Binary Logic5/1 -> Out6/1
  Binary Logic6/1 -> Out7/1
  Binary Logic7/1 -> Out8/1
  Binary Logic8/1 -> Out9/1
  Binary Logic9/1 -> Out10/1
  Binary Logic15/1 -> Out16/1
  Binary Logic14/1 -> Out15/1
  Binary Logic13/1 -> Out14/1
  Binary Logic12/1 -> Out13/1
  Binary Logic11/1 -> Out12/1
  Binary Logic10/1 -> Out11/1

== system aes_impl_decrypt_smc/Round17/Subsystem8 ==
  In1 : Inport
  In2 : Inport  Port=2
  In3 : Inport  Port=3
  In4 : Inport  Port=4
  In5 : Inport  Port=5
  In6 : Inport  Port=6
  In7 : Inport  Port=7
  In8 : Inport  Port=8
  In9 : Inport  Port=9
  In10 : Inport  Port=10
  In11 : Inport  Port=11
  In12 : Inport  Port=12
  In13 : Inport  Port=13
  In14 : Inport  Port=14
  In15 : Inport  Port=15
  In16 : Inport  Port=16
  Subsystem : Subsystem
  Subsystem1 : Subsystem
  Subsystem2 : Subsystem
  Subsystem3 : Subsystem
  Subsystem4 : Subsystem
  Subsystem5 : Subsystem
  Subsystem6 : Subsystem
  Subsystem7 : Subsystem
  Subsystem8 : Subsystem
  Out1 : Outport
  Out2 : Outport  Port=2
  Out3 : Outport  Port=3
  Out4 : Outport  Port=4
  Out5 : Outport  Port=5
  Out6 : Outport  Port=6
  Out7 : Outport  Port=7
  Out8 : Outport  Port=8
  Out9 : Outport  Port=9
  Out10 : Outport  Port=10
  Out11 : Outport  Port=11
  Out12 : Outport  Port=12
  Out13 : Outport  Port=13
  Out14 : Outport  Port=14
  Out15 : Outport  Port=15
  Out16 : Outport  Port=16
  wires:
  Subsystem4/3(Out3) -> Out3/1
  Subsystem4/4(Out4) -> Out4/1
  Subsystem1/1(Out1) -> Out5/1
  Subsystem1/2(Out2) -> Out6/1
  Subsystem1/3(Out3) -> Out7/1
  Subsystem1/4(Out4) -> Out8/1
  Subsystem2/3(Out3) -> Out11/1
  Subsystem2/2(Out2) -> Out10/1
  Subsystem2/1(Out1) -> Out9/1
  Subsystem2/4(Out4) -> Out12/1
  Subsystem3/3(Out3) -> Out15/1
  Subsystem3/2(Out2) -> Out14/1
  Subsystem3/1(Out1) -> Out13/1
  Subsystem/1(Out1) -> Subsystem4/1(In1)
  Subsystem/2(Out2) -> Subsystem4/2(In2)
  Subsystem/3(Out3) -> Subsystem4/3(In3)
  Subsystem/4(Out4) -> Subsystem4/4(In4)
  Subsystem/5(Out5) -> Subsystem1/1(In1)
  Subsystem/6(Out6) -> Subsystem1/2(In2)
  Subsystem/7(Out7) -> Subsystem1/3(In3)
  Subsystem/8(Out8) -> Subsystem1/4(In4)
  Subsystem/9(Out9) -> Subsystem2/1(In1)
  Subsystem/10(Out10) -> Subsystem2/2(In2)
  Subsystem/11(Out11) -> Subsystem2/3(In3)
  Subsystem/12(Out12) -> Subsystem2/4(In4)
  Subsystem/14(Out14) -> Subsystem3/2(In2)
  Subsystem4/1(Out1) -> Out1/1
  Subsystem4/2(Out2) -> Out2/1
  Subsystem3/4(Out4) -> Out16/1
  Subsystem/13(Out13) -> Subsystem3/1(In1)
  Subsystem/15(Out15) -> Subsystem3/3(In3)
  Subsystem/16(Out16) -> Subsystem3/4(In4)
  Subsystem5/2(Out18) -> Subsystem/2(In2)
  Subsystem5/1(Out17) -> Subsystem/1(In1)
  Subsystem5/3(Out19) -> Subsystem/3(In3)
  Subsystem5/4(Out20) -> Subsystem/4(In4)
  In1/1 -> Subsystem5/1(In17)
  In2/1 -> Subsystem5/2(In18)
  In3/1 -> Subsystem5/3(In19)
  In4/1 -> Subsystem5/4(In20)
  Subsystem6/2(Out18) -> Subsystem/6(In6)
  Subsystem6/1(Out17) -> Subsystem/5(In5)
  Subsystem6/3(Out19) -> Subsystem/7(In7)
  Subsystem6/4(Out20) -> Subsystem/8(In8)
  In5/1 -> Subsystem6/1(In17)
  In6/1 -> Subsystem6/2(In18)
  In7/1 -> Subsystem6/3(In19)
  In8/1 -> Subsystem6/4(In20)
  Subsystem7/2(Out18) -> Subsystem/10(In10)
  Subsystem7/1(Out17) -> Subsystem/9(In9)
  Subsystem7/3(Out19) -> Subsystem/11(In11)
  Subsystem7/4(Out20) -> Subsystem/12(In12)
  In9/1 -> Subsystem7/1(In17)
  In10/1 -> Subsystem7/2(In18)
  In11/1 -> Subsystem7/3(In19)
  In12/1 -> Subsystem7/4(In20)
  Subsystem8/2(Out18) -> Subsystem/14(In14)
  Subsystem8/1(Out17) -> Subsystem/13(In13)
  Subsystem8/3(Out19) -> Subsystem/15(In15)
  Subsystem8/4(Out20) -> Subsystem/16(In16)
  In13/1 -> Subsystem8/1(In17)
  In14/1 -> Subsystem8/2(In18)
  In15/1 -> Subsystem8/3(In19)
  In16/1 -> Subsystem8/4(In20)

== system aes_impl_decrypt_smc/Round18/Subsystem ==
  In1 : Inport
  In2 : Inport  Port=2
  In3 : Inport  Port=3
  In4 : Inport  Port=4
  In5 : Inport  Port=5
  In6 : Inport  Port=6
  In7 : Inport  Port=7
  In8 : Inport  Port=8
  In9 : Inport  Port=9
  In10 : Inport  Port=10
  In11 : Inport  Port=11
  In12 : Inport  Port=12
  In13 : Inport  Port=13
  In14 : Inport  Port=14
  In15 : Inport  Port=15
  In16 : Inport  Port=16
  In17 : Inport  Port=17
  In18 : Inport  Port=18
  In19 : Inport  Port=19
  In20 : Inport  Port=20
  In21 : Inport  Port=21
  In22 : Inport  Port=22
  In23 : Inport  Port=23
  In24 : Inport  Port=24
  In25 : Inport  Port=25
  In26 : Inport  Port=26
  In27 : Inport  Port=27
  In28 : Inport  Port=28
  In29 : Inport  Port=29
  In30 : Inport  Port=30
  In31 : Inport  Port=31
  In32 : Inport  Port=32
  Binary Logic{,1..15} (16 alike) : shlslibv1/Math Functions/Binary Logic  syn_binlog_exp=a^b  synBlockType=primitive  synLatency=0  synBlockId=13
  Out1 : Outport
  Out2 : Outport  Port=2
  Out3 : Outport  Port=3
  Out4 : Outport  Port=4
  Out5 : Outport  Port=5
  Out6 : Outport  Port=6
  Out7 : Outport  Port=7
  Out8 : Outport  Port=8
  Out9 : Outport  Port=9
  Out10 : Outport  Port=10
  Out11 : Outport  Port=11
  Out12 : Outport  Port=12
  Out13 : Outport  Port=13
  Out14 : Outport  Port=14
  Out15 : Outport  Port=15
  Out16 : Outport  Port=16
  wires:
  In9/1 -> Binary Logic8/1
  In11/1 -> Binary Logic10/1
  In8/1 -> Binary Logic7/1
  In16/1 -> Binary Logic15/1
  In3/1 -> Binary Logic2/1
  In12/1 -> Binary Logic11/1
  In10/1 -> Binary Logic9/1
  In13/1 -> Binary Logic12/1
  In15/1 -> Binary Logic14/1
  In14/1 -> Binary Logic13/1
  In7/1 -> Binary Logic6/1
  In6/1 -> Binary Logic5/1
  Binary Logic/1 -> Out1/1
  In4/1 -> Binary Logic3/1
  In5/1 -> Binary Logic4/1
  In2/1 -> Binary Logic1/1
  In18/1 -> Binary Logic1/2
  In19/1 -> Binary Logic2/2
  In20/1 -> Binary Logic3/2
  In21/1 -> Binary Logic4/2
  In22/1 -> Binary Logic5/2
  In23/1 -> Binary Logic6/2
  In24/1 -> Binary Logic7/2
  In25/1 -> Binary Logic8/2
  In26/1 -> Binary Logic9/2
  In27/1 -> Binary Logic10/2
  In28/1 -> Binary Logic11/2
  In29/1 -> Binary Logic12/2
  In30/1 -> Binary Logic13/2
  In31/1 -> Binary Logic14/2
  In32/1 -> Binary Logic15/2
  In1/1 -> Binary Logic/1
  In17/1 -> Binary Logic/2
  Binary Logic1/1 -> Out2/1
  Binary Logic2/1 -> Out3/1
  Binary Logic3/1 -> Out4/1
  Binary Logic4/1 -> Out5/1
  Binary Logic5/1 -> Out6/1
  Binary Logic6/1 -> Out7/1
  Binary Logic7/1 -> Out8/1
  Binary Logic8/1 -> Out9/1
  Binary Logic9/1 -> Out10/1
  Binary Logic15/1 -> Out16/1
  Binary Logic14/1 -> Out15/1
  Binary Logic13/1 -> Out14/1
  Binary Logic12/1 -> Out13/1
  Binary Logic11/1 -> Out12/1
  Binary Logic10/1 -> Out11/1

== system aes_impl_decrypt_smc/Round18/Subsystem8 ==
  In1 : Inport
  In2 : Inport  Port=2
  In3 : Inport  Port=3
  In4 : Inport  Port=4
  In5 : Inport  Port=5
  In6 : Inport  Port=6
  In7 : Inport  Port=7
  In8 : Inport  Port=8
  In9 : Inport  Port=9
  In10 : Inport  Port=10
  In11 : Inport  Port=11
  In12 : Inport  Port=12
  In13 : Inport  Port=13
  In14 : Inport  Port=14
  In15 : Inport  Port=15
  In16 : Inport  Port=16
  Subsystem : Subsystem
  Subsystem1 : Subsystem
  Subsystem2 : Subsystem
  Subsystem3 : Subsystem
  Subsystem4 : Subsystem
  Subsystem5 : Subsystem
  Subsystem6 : Subsystem
  Subsystem7 : Subsystem
  Subsystem8 : Subsystem
  Out1 : Outport
  Out2 : Outport  Port=2
  Out3 : Outport  Port=3
  Out4 : Outport  Port=4
  Out5 : Outport  Port=5
  Out6 : Outport  Port=6
  Out7 : Outport  Port=7
  Out8 : Outport  Port=8
  Out9 : Outport  Port=9
  Out10 : Outport  Port=10
  Out11 : Outport  Port=11
  Out12 : Outport  Port=12
  Out13 : Outport  Port=13
  Out14 : Outport  Port=14
  Out15 : Outport  Port=15
  Out16 : Outport  Port=16
  wires:
  Subsystem4/3(Out3) -> Out3/1
  Subsystem4/4(Out4) -> Out4/1
  Subsystem1/1(Out1) -> Out5/1
  Subsystem1/2(Out2) -> Out6/1
  Subsystem1/3(Out3) -> Out7/1
  Subsystem1/4(Out4) -> Out8/1
  Subsystem2/3(Out3) -> Out11/1
  Subsystem2/2(Out2) -> Out10/1
  Subsystem2/1(Out1) -> Out9/1
  Subsystem2/4(Out4) -> Out12/1
  Subsystem3/3(Out3) -> Out15/1
  Subsystem3/2(Out2) -> Out14/1
  Subsystem3/1(Out1) -> Out13/1
  Subsystem/1(Out1) -> Subsystem4/1(In1)
  Subsystem/2(Out2) -> Subsystem4/2(In2)
  Subsystem/3(Out3) -> Subsystem4/3(In3)
  Subsystem/4(Out4) -> Subsystem4/4(In4)
  Subsystem/5(Out5) -> Subsystem1/1(In1)
  Subsystem/6(Out6) -> Subsystem1/2(In2)
  Subsystem/7(Out7) -> Subsystem1/3(In3)
  Subsystem/8(Out8) -> Subsystem1/4(In4)
  Subsystem/9(Out9) -> Subsystem2/1(In1)
  Subsystem/10(Out10) -> Subsystem2/2(In2)
  Subsystem/11(Out11) -> Subsystem2/3(In3)
  Subsystem/12(Out12) -> Subsystem2/4(In4)
  Subsystem/14(Out14) -> Subsystem3/2(In2)
  Subsystem4/1(Out1) -> Out1/1
  Subsystem4/2(Out2) -> Out2/1
  Subsystem3/4(Out4) -> Out16/1
  Subsystem/13(Out13) -> Subsystem3/1(In1)
  Subsystem/15(Out15) -> Subsystem3/3(In3)
  Subsystem/16(Out16) -> Subsystem3/4(In4)
  Subsystem5/2(Out18) -> Subsystem/2(In2)
  Subsystem5/1(Out17) -> Subsystem/1(In1)
  Subsystem5/3(Out19) -> Subsystem/3(In3)
  Subsystem5/4(Out20) -> Subsystem/4(In4)
  In1/1 -> Subsystem5/1(In17)
  In2/1 -> Subsystem5/2(In18)
  In3/1 -> Subsystem5/3(In19)
  In4/1 -> Subsystem5/4(In20)
  Subsystem6/2(Out18) -> Subsystem/6(In6)
  Subsystem6/1(Out17) -> Subsystem/5(In5)
  Subsystem6/3(Out19) -> Subsystem/7(In7)
  Subsystem6/4(Out20) -> Subsystem/8(In8)
  In5/1 -> Subsystem6/1(In17)
  In6/1 -> Subsystem6/2(In18)
  In7/1 -> Subsystem6/3(In19)
  In8/1 -> Subsystem6/4(In20)
  Subsystem7/2(Out18) -> Subsystem/10(In10)
  Subsystem7/1(Out17) -> Subsystem/9(In9)
  Subsystem7/3(Out19) -> Subsystem/11(In11)
  Subsystem7/4(Out20) -> Subsystem/12(In12)
  In9/1 -> Subsystem7/1(In17)
  In10/1 -> Subsystem7/2(In18)
  In11/1 -> Subsystem7/3(In19)
  In12/1 -> Subsystem7/4(In20)
  Subsystem8/2(Out18) -> Subsystem/14(In14)
  Subsystem8/1(Out17) -> Subsystem/13(In13)
  Subsystem8/3(Out19) -> Subsystem/15(In15)
  Subsystem8/4(Out20) -> Subsystem/16(In16)
  In13/1 -> Subsystem8/1(In17)
  In14/1 -> Subsystem8/2(In18)
  In15/1 -> Subsystem8/3(In19)
  In16/1 -> Subsystem8/4(In20)

== system aes_impl_decrypt_smc/Round19/Subsystem ==
  In1 : Inport
  In2 : Inport  Port=2
  In3 : Inport  Port=3
  In4 : Inport  Port=4
  In5 : Inport  Port=5
  In6 : Inport  Port=6
  In7 : Inport  Port=7
  In8 : Inport  Port=8
  In9 : Inport  Port=9
  In10 : Inport  Port=10
  In11 : Inport  Port=11
  In12 : Inport  Port=12
  In13 : Inport  Port=13
  In14 : Inport  Port=14
  In15 : Inport  Port=15
  In16 : Inport  Port=16
  In17 : Inport  Port=17
  In18 : Inport  Port=18
  In19 : Inport  Port=19
  In20 : Inport  Port=20
  In21 : Inport  Port=21
  In22 : Inport  Port=22
  In23 : Inport  Port=23
  In24 : Inport  Port=24
  In25 : Inport  Port=25
  In26 : Inport  Port=26
  In27 : Inport  Port=27
  In28 : Inport  Port=28
  In29 : Inport  Port=29
  In30 : Inport  Port=30
  In31 : Inport  Port=31
  In32 : Inport  Port=32
  Binary Logic{,1..15} (16 alike) : shlslibv1/Math Functions/Binary Logic  syn_binlog_exp=a^b  synBlockType=primitive  synLatency=0  synBlockId=13
  Out1 : Outport
  Out2 : Outport  Port=2
  Out3 : Outport  Port=3
  Out4 : Outport  Port=4
  Out5 : Outport  Port=5
  Out6 : Outport  Port=6
  Out7 : Outport  Port=7
  Out8 : Outport  Port=8
  Out9 : Outport  Port=9
  Out10 : Outport  Port=10
  Out11 : Outport  Port=11
  Out12 : Outport  Port=12
  Out13 : Outport  Port=13
  Out14 : Outport  Port=14
  Out15 : Outport  Port=15
  Out16 : Outport  Port=16
  wires:
  In9/1 -> Binary Logic8/1
  In11/1 -> Binary Logic10/1
  In8/1 -> Binary Logic7/1
  In16/1 -> Binary Logic15/1
  In3/1 -> Binary Logic2/1
  In12/1 -> Binary Logic11/1
  In10/1 -> Binary Logic9/1
  In13/1 -> Binary Logic12/1
  In15/1 -> Binary Logic14/1
  In14/1 -> Binary Logic13/1
  In7/1 -> Binary Logic6/1
  In6/1 -> Binary Logic5/1
  Binary Logic/1 -> Out1/1
  In4/1 -> Binary Logic3/1
  In5/1 -> Binary Logic4/1
  In2/1 -> Binary Logic1/1
  In18/1 -> Binary Logic1/2
  In19/1 -> Binary Logic2/2
  In20/1 -> Binary Logic3/2
  In21/1 -> Binary Logic4/2
  In22/1 -> Binary Logic5/2
  In23/1 -> Binary Logic6/2
  In24/1 -> Binary Logic7/2
  In25/1 -> Binary Logic8/2
  In26/1 -> Binary Logic9/2
  In27/1 -> Binary Logic10/2
  In28/1 -> Binary Logic11/2
  In29/1 -> Binary Logic12/2
  In30/1 -> Binary Logic13/2
  In31/1 -> Binary Logic14/2
  In32/1 -> Binary Logic15/2
  In1/1 -> Binary Logic/1
  In17/1 -> Binary Logic/2
  Binary Logic1/1 -> Out2/1
  Binary Logic2/1 -> Out3/1
  Binary Logic3/1 -> Out4/1
  Binary Logic4/1 -> Out5/1
  Binary Logic5/1 -> Out6/1
  Binary Logic6/1 -> Out7/1
  Binary Logic7/1 -> Out8/1
  Binary Logic8/1 -> Out9/1
  Binary Logic9/1 -> Out10/1
  Binary Logic15/1 -> Out16/1
  Binary Logic14/1 -> Out15/1
  Binary Logic13/1 -> Out14/1
  Binary Logic12/1 -> Out13/1
  Binary Logic11/1 -> Out12/1
  Binary Logic10/1 -> Out11/1

== system aes_impl_decrypt_smc/Round19/Subsystem8 ==
  In1 : Inport
  In2 : Inport  Port=2
  In3 : Inport  Port=3
  In4 : Inport  Port=4
  In5 : Inport  Port=5
  In6 : Inport  Port=6
  In7 : Inport  Port=7
  In8 : Inport  Port=8
  In9 : Inport  Port=9
  In10 : Inport  Port=10
  In11 : Inport  Port=11
  In12 : Inport  Port=12
  In13 : Inport  Port=13
  In14 : Inport  Port=14
  In15 : Inport  Port=15
  In16 : Inport  Port=16
  Subsystem : Subsystem
  Subsystem1 : Subsystem
  Subsystem2 : Subsystem
  Subsystem3 : Subsystem
  Subsystem4 : Subsystem
  Subsystem5 : Subsystem
  Subsystem6 : Subsystem
  Subsystem7 : Subsystem
  Subsystem8 : Subsystem
  Out1 : Outport
  Out2 : Outport  Port=2
  Out3 : Outport  Port=3
  Out4 : Outport  Port=4
  Out5 : Outport  Port=5
  Out6 : Outport  Port=6
  Out7 : Outport  Port=7
  Out8 : Outport  Port=8
  Out9 : Outport  Port=9
  Out10 : Outport  Port=10
  Out11 : Outport  Port=11
  Out12 : Outport  Port=12
  Out13 : Outport  Port=13
  Out14 : Outport  Port=14
  Out15 : Outport  Port=15
  Out16 : Outport  Port=16
  wires:
  Subsystem4/3(Out3) -> Out3/1
  Subsystem4/4(Out4) -> Out4/1
  Subsystem1/1(Out1) -> Out5/1
  Subsystem1/2(Out2) -> Out6/1
  Subsystem1/3(Out3) -> Out7/1
  Subsystem1/4(Out4) -> Out8/1
  Subsystem2/3(Out3) -> Out11/1
  Subsystem2/2(Out2) -> Out10/1
  Subsystem2/1(Out1) -> Out9/1
  Subsystem2/4(Out4) -> Out12/1
  Subsystem3/3(Out3) -> Out15/1
  Subsystem3/2(Out2) -> Out14/1
  Subsystem3/1(Out1) -> Out13/1
  Subsystem/1(Out1) -> Subsystem4/1(In1)
  Subsystem/2(Out2) -> Subsystem4/2(In2)
  Subsystem/3(Out3) -> Subsystem4/3(In3)
  Subsystem/4(Out4) -> Subsystem4/4(In4)
  Subsystem/5(Out5) -> Subsystem1/1(In1)
  Subsystem/6(Out6) -> Subsystem1/2(In2)
  Subsystem/7(Out7) -> Subsystem1/3(In3)
  Subsystem/8(Out8) -> Subsystem1/4(In4)
  Subsystem/9(Out9) -> Subsystem2/1(In1)
  Subsystem/10(Out10) -> Subsystem2/2(In2)
  Subsystem/11(Out11) -> Subsystem2/3(In3)
  Subsystem/12(Out12) -> Subsystem2/4(In4)
  Subsystem/14(Out14) -> Subsystem3/2(In2)
  Subsystem4/1(Out1) -> Out1/1
  Subsystem4/2(Out2) -> Out2/1
  Subsystem3/4(Out4) -> Out16/1
  Subsystem/13(Out13) -> Subsystem3/1(In1)
  Subsystem/15(Out15) -> Subsystem3/3(In3)
  Subsystem/16(Out16) -> Subsystem3/4(In4)
  Subsystem5/2(Out18) -> Subsystem/2(In2)
  Subsystem5/1(Out17) -> Subsystem/1(In1)
  Subsystem5/3(Out19) -> Subsystem/3(In3)
  Subsystem5/4(Out20) -> Subsystem/4(In4)
  In1/1 -> Subsystem5/1(In17)
  In2/1 -> Subsystem5/2(In18)
  In3/1 -> Subsystem5/3(In19)
  In4/1 -> Subsystem5/4(In20)
  Subsystem6/2(Out18) -> Subsystem/6(In6)
  Subsystem6/1(Out17) -> Subsystem/5(In5)
  Subsystem6/3(Out19) -> Subsystem/7(In7)
  Subsystem6/4(Out20) -> Subsystem/8(In8)
  In5/1 -> Subsystem6/1(In17)
  In6/1 -> Subsystem6/2(In18)
  In7/1 -> Subsystem6/3(In19)
  In8/1 -> Subsystem6/4(In20)
  Subsystem7/2(Out18) -> Subsystem/10(In10)
  Subsystem7/1(Out17) -> Subsystem/9(In9)
  Subsystem7/3(Out19) -> Subsystem/11(In11)
  Subsystem7/4(Out20) -> Subsystem/12(In12)
  In9/1 -> Subsystem7/1(In17)
  In10/1 -> Subsystem7/2(In18)
  In11/1 -> Subsystem7/3(In19)
  In12/1 -> Subsystem7/4(In20)
  Subsystem8/2(Out18) -> Subsystem/14(In14)
  Subsystem8/1(Out17) -> Subsystem/13(In13)
  Subsystem8/3(Out19) -> Subsystem/15(In15)
  Subsystem8/4(Out20) -> Subsystem/16(In16)
  In13/1 -> Subsystem8/1(In17)
  In14/1 -> Subsystem8/2(In18)
  In15/1 -> Subsystem8/3(In19)
  In16/1 -> Subsystem8/4(In20)

== system aes_impl_decrypt_smc/Round2/Key1 ==
  In1 : Inport
  In2 : Inport  Port=2
  In3 : Inport  Port=3
  In4 : Inport  Port=4
  In5 : Inport  Port=5
  In6 : Inport  Port=6
  In7 : Inport  Port=7
  In8 : Inport  Port=8
  In9 : Inport  Port=9
  In10 : Inport  Port=10
  In11 : Inport  Port=11
  In12 : Inport  Port=12
  In13 : Inport  Port=13
  In14 : Inport  Port=14
  In15 : Inport  Port=15
  In16 : Inport  Port=16
  Keygen1 : Subsystem
  Keygen2 : Subsystem
  Keygen3 : Subsystem
  Keygen4 : Subsystem
  Out1 : Outport
  Out2 : Outport  Port=2
  Out3 : Outport  Port=3
  Out4 : Outport  Port=4
  Out5 : Outport  Port=5
  Out6 : Outport  Port=6
  Out7 : Outport  Port=7
  Out8 : Outport  Port=8
  Out9 : Outport  Port=9
  Out10 : Outport  Port=10
  Out11 : Outport  Port=11
  Out12 : Outport  Port=12
  Out13 : Outport  Port=13
  Out14 : Outport  Port=14
  Out15 : Outport  Port=15
  Out16 : Outport  Port=16
  wires:
  Keygen1/3(Out3) -> Out3/1, Keygen2/3(In3)
  In2/1 -> Keygen1/2(In2)
  Keygen3/2(Out2) -> Keygen4/2(In2), Out10/1
  Keygen2/4(Out4) -> Keygen3/4(In4), Out8/1
  Keygen4/4(Out4) -> Out16/1
  Keygen4/2(Out2) -> Out14/1
  In3/1 -> Keygen1/3(In3)
  Keygen2/2(Out2) -> Keygen3/2(In2), Out6/1
  Keygen2/1(Out1) -> Keygen3/1(In1), Out5/1
  In1/1 -> Keygen1/1(In1)
  Keygen4/1(Out1) -> Out13/1
  In4/1 -> Keygen1/4(In4)
  Keygen3/4(Out4) -> Keygen4/4(In4), Out12/1
  Keygen1/4(Out4) -> Keygen2/4(In4), Out4/1
  Keygen2/3(Out3) -> Keygen3/3(In3), Out7/1
  Keygen1/2(Out2) -> Keygen2/2(In2), Out2/1
  Keygen1/1(Out1) -> Keygen2/1(In1), Out1/1
  Keygen4/3(Out3) -> Out15/1
  Keygen3/1(Out1) -> Keygen4/1(In1), Out9/1
  Keygen3/3(Out3) -> Keygen4/3(In3), Out11/1
  In5/1 -> Keygen2/5(In5)
  In7/1 -> Keygen2/7(In7)
  In8/1 -> Keygen2/8(In8)
  In6/1 -> Keygen2/6(In6)
  In9/1 -> Keygen3/5(In5)
  In10/1 -> Keygen3/6(In6)
  In11/1 -> Keygen3/7(In7)
  In12/1 -> Keygen3/8(In8)
  In13/1 -> Keygen4/5(In5), Keygen1/5(In5)
  In14/1 -> Keygen4/6(In6), Keygen1/6(In6)
  In15/1 -> Keygen4/7(In7), Keygen1/7(In7)
  In16/1 -> Keygen4/8(In8), Keygen1/8(In8)
